simulink model "ROS_Control_for_ModularBus_cs"  (R2023a)
settings: Solver=ode5  StartTime=0.0  StopTime=inf  FixedStep=1/1000  RelTol=1e-3
PreLoadFcn:
  | mbxruntime.callbacks.PreLoadFcn(bdroot);
PostLoadFcn:
  | mbxruntime.callbacks.PostLoadFcn(bdroot);
InitFcn:
  | mbxruntime.callbacks.InitFcn(bdroot);
StartFcn:
  | mbxruntime.callbacks.StartFcn(bdroot);
StopFcn:
  | mbxruntime.callbacks.StopFcn(bdroot);
model workspace: external: MAT-File .\ROS_Control_for_ModularBus_cs_hws.mat (data not in the file)
values from neighbouring files (symbols this model uses):
  c_factor = 43.75    [emplanner_init.m]
  cf = -64276.3    [emplanner_init.m]
  cr = -64276.3    [emplanner_init.m]
  host_x_init = 0    [emplanner_init.m]
  host_y_init = 0    [emplanner_init.m]
  KD_PID_distance = 0.05    [emplanner_init.m]
  KD_PID_speed = 0.01    [emplanner_init.m]
  KI_PID_distance = 0.01    [emplanner_init.m]
  KI_PID_speed = 0.02    [emplanner_init.m]
  KP_PID_distance = 0.1    [emplanner_init.m]
  KP_PID_speed = 0.2    [emplanner_init.m]
  la = 0.5989    [emplanner_init.m]
  lb = 1.1979-0.5989    (= 0.599)    [emplanner_init.m]
  LQR_K1 = k(:,1)'    [emplanner_init.m]
  LQR_K2 = k(:,2)'    [emplanner_init.m]
  LQR_K3 = k(:,3)'    [emplanner_init.m]
  LQR_K4 = k(:,4)'    [emplanner_init.m]
  m = 375.8    [emplanner_init.m]
  vx_break_point = zeros(1,5000)    [emplanner_init.m]
undefined symbols (not defined in the file or in its folder): aubr, DiscIntNeverNeededParam, mbxruntime, rack_displacement, right_wheel_ground, ROS_Control_for_ModularBus_cs_018403cc6703814a, ROS_Control_for_ModularBus_cs_040a1db8f50ecaa9, ROS_Control_for_ModularBus_cs_059bdebef014cf08, ROS_Control_for_ModularBus_cs_0c250e3b2f70afe8, ROS_Control_for_ModularBus_cs_1665011a38ab79d0, ROS_Control_for_ModularBus_cs_17829354c8add7a7, ROS_Control_for_ModularBus_cs_19e468234ea448bc, ROS_Control_for_ModularBus_cs_27ae15b290bbaf4d, ROS_Control_for_ModularBus_cs_27eba31aa8e5b642, ROS_Control_for_ModularBus_cs_297ea4fdef143881, ROS_Control_for_ModularBus_cs_2b4063ae14d997a3, ROS_Control_for_ModularBus_cs_2c04773b04fadd8f, ROS_Control_for_ModularBus_cs_346eb3b7c82070b1, ROS_Control_for_ModularBus_cs_3f31df18790d0857, ROS_Control_for_ModularBus_cs_6035221df40a0068, ROS_Control_for_ModularBus_cs_605cc8a35cf1fbee, ROS_Control_for_ModularBus_cs_60f7501961f824af, ROS_Control_for_ModularBus_cs_6afca23e567ce192, ROS_Control_for_ModularBus_cs_722492775f672945, ROS_Control_for_ModularBus_cs_722a0847cfabd36b, ROS_Control_for_ModularBus_cs_739dd6601d79d035, ROS_Control_for_ModularBus_cs_7b4de5d0566f485f, ROS_Control_for_ModularBus_cs_7b8949829b72752d, ROS_Control_for_ModularBus_cs_82c4092e07cd044c, ROS_Control_for_ModularBus_cs_89fd7107669e07b9, ROS_Control_for_ModularBus_cs_8a6008cabae637b7, ROS_Control_for_ModularBus_cs_96f82902791ad622, ROS_Control_for_ModularBus_cs_9811c31d07ac9f2b, ROS_Control_for_ModularBus_cs_9ce2872cbf4b1b23, ROS_Control_for_ModularBus_cs_9d5a7f5c2803ee13, ROS_Control_for_ModularBus_cs_a623587393f1eaea, ROS_Control_for_ModularBus_cs_a7debeb2acd4f548, ROS_Control_for_ModularBus_cs_aa8fbbb7fdfec12a, ROS_Control_for_ModularBus_cs_ac425023a351a898, ROS_Control_for_ModularBus_cs_b3d4de7570946bb3, ROS_Control_for_ModularBus_cs_b771f0870c594399, ROS_Control_for_ModularBus_cs_bac30ea3d3bfebea, ROS_Control_for_ModularBus_cs_bd760ea296acac74, ROS_Control_for_ModularBus_cs_be4fa55e319672a9, ROS_Control_for_ModularBus_cs_c84eac9215852fa9, ROS_Control_for_ModularBus_cs_c9fa3144fa1cc4e3, ROS_Control_for_ModularBus_cs_caf32c655ee9484b, ROS_Control_for_ModularBus_cs_d133acedd44eb8df, ROS_Control_for_ModularBus_cs_d4613310abe0108f, ROS_Control_for_ModularBus_cs_dac9c98002987d8c, ROS_Control_for_ModularBus_cs_db335108f6550d72, ROS_Control_for_ModularBus_cs_dc60765170b71665, ROS_Control_for_ModularBus_cs_e0417f4e6fa341f5, ROS_Control_for_ModularBus_cs_e34124fd4d75bbae, ROS_Control_for_ModularBus_cs_e3fac3581a45c347, ROS_Control_for_ModularBus_cs_e5e08783dc4f74d5, ROS_Control_for_ModularBus_cs_ea1cf1e0b24b8a39, ROS_Control_for_ModularBus_cs_fa2a9ba8914f8ed6, ROS_Control_for_ModularBus_cs_faa52b96bad252bf, tablebr ... (+1)
libraries: PreScanSimulinkLibrary x18, robotlib x2, Solver_SF x1
(part 5 of 5)

== system ROS_Control_for_ModularBus_cs/Box_4/SELF_Demux/compas converter/cart2compas ==
  Angle [deg] : Inport
  Constant : Constant  Value=90
  Constant1 : Constant  Value=360
  Gain : Gain  Gain=1/360
  Gain1 : Gain  Gain=360
  Gain2 : Gain  Gain=-1
  Rounding Function : Rounding
  Sum : Sum  Inputs=|-+
  Sum1 : Sum  Inputs=-+|
  Sum2 : Sum  Inputs=++|
  heading [deg] : Outport
  wires:
  Gain/1 -> Rounding Function/1
  Rounding Function/1 -> Gain1/1
  Gain1/1 -> Sum/1
  Angle [deg]/1 -> Sum1/2
  Sum/1 -> Gain2/1
  Sum1/1 -> Gain/1, Sum/2
  Constant/1 -> Sum1/1
  Gain2/1 -> Sum2/2
  Constant1/1 -> Sum2/1
  Sum2/1 -> heading [deg]/1

== system ROS_Control_for_ModularBus_cs/Box_5/SELF_Demux/compas converter/cart2compas ==
  Angle [deg] : Inport
  Constant : Constant  Value=90
  Constant1 : Constant  Value=360
  Gain : Gain  Gain=1/360
  Gain1 : Gain  Gain=360
  Gain2 : Gain  Gain=-1
  Rounding Function : Rounding
  Sum : Sum  Inputs=|-+
  Sum1 : Sum  Inputs=-+|
  Sum2 : Sum  Inputs=++|
  heading [deg] : Outport
  wires:
  Gain/1 -> Rounding Function/1
  Rounding Function/1 -> Gain1/1
  Gain1/1 -> Sum/1
  Angle [deg]/1 -> Sum1/2
  Sum/1 -> Gain2/1
  Sum1/1 -> Gain/1, Sum/2
  Constant/1 -> Sum1/1
  Gain2/1 -> Sum2/2
  Constant1/1 -> Sum2/1
  Sum2/1 -> heading [deg]/1

== system ROS_Control_for_ModularBus_cs/Box_6/SELF_Demux/compas converter/cart2compas ==
  Angle [deg] : Inport
  Constant : Constant  Value=90
  Constant1 : Constant  Value=360
  Gain : Gain  Gain=1/360
  Gain1 : Gain  Gain=360
  Gain2 : Gain  Gain=-1
  Rounding Function : Rounding
  Sum : Sum  Inputs=|-+
  Sum1 : Sum  Inputs=-+|
  Sum2 : Sum  Inputs=++|
  heading [deg] : Outport
  wires:
  Gain/1 -> Rounding Function/1
  Rounding Function/1 -> Gain1/1
  Gain1/1 -> Sum/1
  Angle [deg]/1 -> Sum1/2
  Sum/1 -> Gain2/1
  Sum1/1 -> Gain/1, Sum/2
  Constant/1 -> Sum1/1
  Gain2/1 -> Sum2/2
  Constant1/1 -> Sum2/1
  Sum2/1 -> heading [deg]/1

== system ROS_Control_for_ModularBus_cs/Box_7/SELF_Demux/compas converter/cart2compas ==
  Angle [deg] : Inport
  Constant : Constant  Value=90
  Constant1 : Constant  Value=360
  Gain : Gain  Gain=1/360
  Gain1 : Gain  Gain=360
  Gain2 : Gain  Gain=-1
  Rounding Function : Rounding
  Sum : Sum  Inputs=|-+
  Sum1 : Sum  Inputs=-+|
  Sum2 : Sum  Inputs=++|
  heading [deg] : Outport
  wires:
  Gain/1 -> Rounding Function/1
  Rounding Function/1 -> Gain1/1
  Gain1/1 -> Sum/1
  Angle [deg]/1 -> Sum1/2
  Sum/1 -> Gain2/1
  Sum1/1 -> Gain/1, Sum/2
  Constant/1 -> Sum1/1
  Gain2/1 -> Sum2/2
  Constant1/1 -> Sum2/1
  Sum2/1 -> heading [deg]/1

== system ROS_Control_for_ModularBus_cs/Box_8/SELF_Demux/compas converter/cart2compas ==
  Angle [deg] : Inport
  Constant : Constant  Value=90
  Constant1 : Constant  Value=360
  Gain : Gain  Gain=1/360
  Gain1 : Gain  Gain=360
  Gain2 : Gain  Gain=-1
  Rounding Function : Rounding
  Sum : Sum  Inputs=|-+
  Sum1 : Sum  Inputs=-+|
  Sum2 : Sum  Inputs=++|
  heading [deg] : Outport
  wires:
  Gain/1 -> Rounding Function/1
  Rounding Function/1 -> Gain1/1
  Gain1/1 -> Sum/1
  Angle [deg]/1 -> Sum1/2
  Sum/1 -> Gain2/1
  Sum1/1 -> Gain/1, Sum/2
  Constant/1 -> Sum1/1
  Gain2/1 -> Sum2/2
  Constant1/1 -> Sum2/1
  Sum2/1 -> heading [deg]/1

== system ROS_Control_for_ModularBus_cs/modular_bus_1/Dynamics_UserSpecified/CarSim2PreScanSTATE/Transformation_SprungMassCarSim2PreScan ==
  In1 : Inport
  Demux : Demux  Outputs=3
  Ini z-position VEHICLE wrt GLOBAL axis system [m] : Constant  Value=z0
  Mux : Mux  Inputs=3
  Sum1 : Sum  Inputs=+-
  Out1 : Outport  VectorParamsAs1DForOutWhenUnconnected=off
  wires:
  Mux/1 -> Out1/1
  Ini z-position VEHICLE wrt GLOBAL axis system [m]/1 -> Sum1/2
  Demux/1 -> Mux/1
  Sum1/1 -> Mux/3
  Demux/3 -> Sum1/1
  Demux/2 -> Mux/2
  In1/1 -> Demux/1

== system ROS_Control_for_ModularBus_cs/modular_bus_1/SELF_Demux/compas converter/cart2compas ==
  Angle [deg] : Inport
  Constant : Constant  Value=90
  Constant1 : Constant  Value=360
  Gain : Gain  Gain=1/360
  Gain1 : Gain  Gain=360
  Gain2 : Gain  Gain=-1
  Rounding Function : Rounding
  Sum : Sum  Inputs=|-+
  Sum1 : Sum  Inputs=-+|
  Sum2 : Sum  Inputs=++|
  heading [deg] : Outport
  wires:
  Gain/1 -> Rounding Function/1
  Rounding Function/1 -> Gain1/1
  Gain1/1 -> Sum/1
  Angle [deg]/1 -> Sum1/2
  Sum/1 -> Gain2/1
  Sum1/1 -> Gain/1, Sum/2
  Constant/1 -> Sum1/1
  Gain2/1 -> Sum2/2
  Constant1/1 -> Sum2/1
  Sum2/1 -> heading [deg]/1

== system ROS_Control_for_ModularBus_cs/modular_bus_1/control module/control main/chassic steering system ==
  LQR_final_angle : Inport
  Constant : Constant  Value=la
  Constant1 : Constant  Value=lb
  Constant17 : Constant  Value=c_factor
  Divide : Product  Inputs=*/
  Gain3 : Gain  Gain=180/pi
  Gain4 : Gain  Gain=360
  MATLAB Function : MATLAB Function  TreatAsAtomicUnit=on
  Saturation : Saturate  UpperLimit=70  LowerLimit=-70
  Saturation1 : Saturate  UpperLimit=1.2217  LowerLimit=-1.2217
  transfer right wheel angle to rack displancement : Lookup_n-D  NumberOfTableDimensions=1  BreakpointsForDimension1=right_wheel_ground  Table=rack_displacement  InternalRulePriority=Speed  RndMeth=Simplest
  lat_steer_sw[deg] : Outport
  wires:
  transfer right wheel angle to rack displancement/1 -> Divide/1
  Constant17/1 -> Divide/2
  Gain4/1 -> lat_steer_sw[deg]/1
  Divide/1 -> Gain4/1
  Saturation/1 -> transfer right wheel angle to rack displancement/1
  Constant/1 -> MATLAB Function/2(la)
  Gain3/1 -> Saturation/1
  Constant1/1 -> MATLAB Function/3(lb)
  LQR_final_angle/1 -> Saturation1/1
  Saturation1/1 -> MATLAB Function/1(u)
  MATLAB Function/1(right_steer) -> Gain3/1

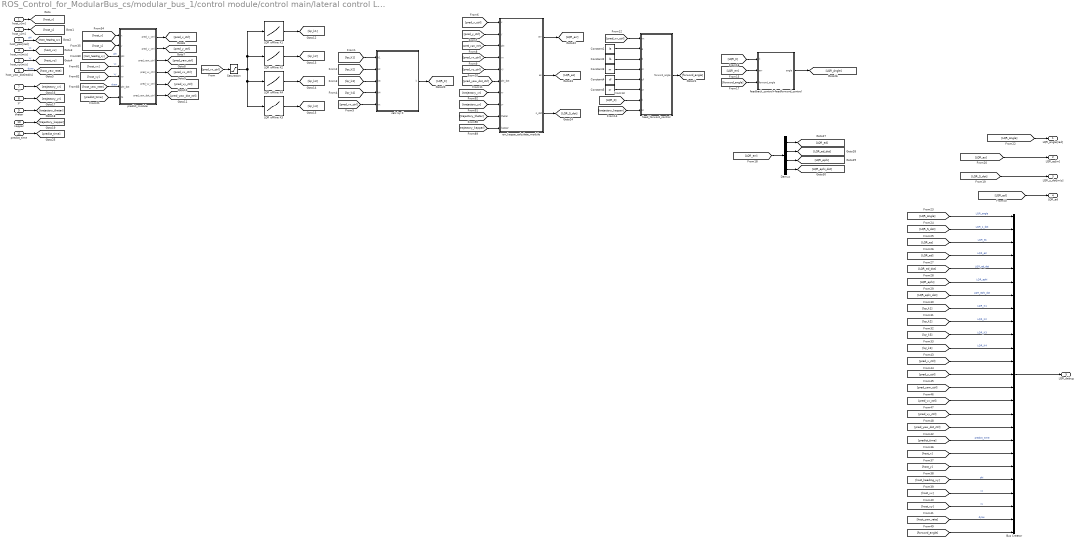
== system ROS_Control_for_ModularBus_cs/modular_bus_1/control module/control main/lateral control LQR ==
  host_x[m] : Inport
  host_y[m] : Inport  Port=2
  host_yaw[rad] : Inport  Port=3
  host_vx[m/s] : Inport  Port=4
  host_vy[m/s] : Inport  Port=5
  host_yaw_dot[rad/s] : Inport  Port=6
  xr : Inport  Port=7
  yr : Inport  Port=8
  thetar : Inport  Port=9
  kappar : Inport  Port=10
  predict_time : Inport  Port=11
  Bus Creator : BusCreator  Inputs=25
  Constant1 : Constant  Value=la
  Constant2 : Constant  Value=lb
  Constant3 : Constant  Value=m
  Constant4 : Constant  Value=cf
  Constant5 : Constant  Value=cr
  Demux : Demux
  LQR offline K1 : Lookup_n-D  NumberOfTableDimensions=1  BreakpointsForDimension1=vx_break_point  Table=LQR_K1  InternalRulePriority=Speed  RndMeth=Simplest
  LQR offline K2 : Lookup_n-D  NumberOfTableDimensions=1  BreakpointsForDimension1=vx_break_point  Table=LQR_K2  InternalRulePriority=Speed  RndMeth=Simplest
  LQR offline K3 : Lookup_n-D  NumberOfTableDimensions=1  BreakpointsForDimension1=vx_break_point  Table=LQR_K3  InternalRulePriority=Speed  RndMeth=Simplest
  LQR offline K4 : Lookup_n-D  NumberOfTableDimensions=1  BreakpointsForDimension1=vx_break_point  Table=LQR_K4  InternalRulePriority=Speed  RndMeth=Simplest
  Saturation : Saturate  UpperLimit=50  LowerLimit=0
  calc lqr K : MATLAB Function  TreatAsAtomicUnit=on
  err_kappa_calculate_module : MATLAB Function  TreatAsAtomicUnit=on
  feed_forword_control : MATLAB Function  TreatAsAtomicUnit=on
  feedback_control+feedforword_control : MATLAB Function  TreatAsAtomicUnit=on
  predict_module : MATLAB Function  TreatAsAtomicUnit=on
  LQR_angle[rad] : Outport  VectorParamsAs1DForOutWhenUnconnected=off
  LQR_es[m] : Outport  Port=2  VectorParamsAs1DForOutWhenUnconnected=off
  LQR_s_dot[m/s] : Outport  Port=3  VectorParamsAs1DForOutWhenUnconnected=off
  LQR_ed : Outport  Port=4  VectorParamsAs1DForOutWhenUnconnected=off
  LQR_debug : Outport  Port=5  VectorParamsAs1DForOutWhenUnconnected=off
  wires:
  [host_vy] -> predict_module/5(vy)  "vy"
  [host_x] -> predict_module/1(x)
  [host_yaw_rate] -> predict_module/6(phi_dot)  "dyaw"
  [host_vx] -> predict_module/4(vx)  "vx"
  [host_y] -> predict_module/2(y)
  [host_heading_xy] -> predict_module/3(phi)  "phi"
  [predict_time] -> predict_module/7(ts)
  host_x[m]/1 -> [host_x]
  host_y[m]/1 -> [host_y]
  host_yaw[rad]/1 -> [host_heading_xy]  "phi"
  host_vx[m/s]/1 -> [host_vx]  "vx"
  host_vy[m/s]/1 -> [host_vy]  "vy"
  host_yaw_dot[rad/s]/1 -> [host_yaw_rate]  "dyaw"
  predict_module/1(pred_x_ctrl) -> [pred_x_ctrl]
  predict_module/2(pred_y_ctrl) -> [pred_y_ctrl]
  predict_module/3(pred_yaw_ctrl) -> [pred_yaw_ctrl]
  predict_module/4(pred_vx_ctrl) -> [pred_vx_ctrl]
  predict_module/5(pred_vy_ctrl) -> [pred_vy_ctrl]
  predict_module/6(pred_yaw_dot_ctrl) -> [pred_yaw_dot_ctrl]
  [pred_vx_ctrl] -> Saturation/1
  LQR offline K1/1 -> [lqr_k1]
  LQR offline K2/1 -> [lqr_k2]
  LQR offline K4/1 -> [lqr_k3]
  LQR offline K3/1 -> [lqr_k4]
  [pred_vx_ctrl] -> calc lqr K/5(vx)
  [lqr_k4] -> calc lqr K/4(k4)
  [lqr_k3] -> calc lqr K/3(k3)
  [lqr_k2] -> calc lqr K/2(k2)
  [lqr_k1] -> calc lqr K/1(k1)
  [pred_x_ctrl] -> err_kappa_calculate_module/1(x)
  [pred_y_ctrl] -> err_kappa_calculate_module/2(y)
  [pred_yaw_ctrl] -> err_kappa_calculate_module/3(phi)
  [pred_vx_ctrl] -> err_kappa_calculate_module/4(vx)
  [pred_vy_ctrl] -> err_kappa_calculate_module/5(vy)
  [pred_yaw_dot_ctrl] -> err_kappa_calculate_module/6(phi_dot)
  xr/1 -> [trajectory_xr]
  yr/1 -> [trajectory_yr]
  thetar/1 -> [trajectory_thetar]
  kappar/1 -> [trajectory_kappar]
  [trajectory_xr] -> err_kappa_calculate_module/7(xr)
  [trajectory_yr] -> err_kappa_calculate_module/8(yr)
  [trajectory_kappar] -> err_kappa_calculate_module/10(kappar)
  [trajectory_thetar] -> err_kappa_calculate_module/9(thetar)
  [pred_vx_ctrl] -> feed_forword_control/1(vx)
  Constant1/1 -> feed_forword_control/2(a)
  Constant2/1 -> feed_forword_control/3(b)
  Constant3/1 -> feed_forword_control/4(m)
  Constant4/1 -> feed_forword_control/5(cf)
  Constant5/1 -> feed_forword_control/6(cr)
  calc lqr K/1(k) -> [LQR_K]
  [LQR_K] -> feed_forword_control/7(k)
  [trajectory_kappar] -> feed_forword_control/8(kr)
  feed_forword_control/1(forword_angle) -> [forword_angle]
  err_kappa_calculate_module/1(err) -> [LQR_err]
  [LQR_err] -> feedback_control+feedforword_control/2(err)
  [LQR_K] -> feedback_control+feedforword_control/1(k)
  [forword_angle] -> feedback_control+feedforword_control/3(forword_angle)
  [LQR_err] -> Demux/1
  err_kappa_calculate_module/2(es) -> [LQR_es]
  err_kappa_calculate_module/3(s_dot) -> [LQR_S_dot]
  [LQR_S_dot] -> LQR_s_dot[m/s]/1
  [LQR_es] -> LQR_es[m]/1
  Saturation/1 -> LQR offline K3/1, LQR offline K4/1, LQR offline K2/1, LQR offline K1/1
  predict_time/1 -> [predict_time]
  Bus Creator/1 -> LQR_debug/1
  feedback_control+feedforword_control/1(angle) -> [LQR_Angle]
  [LQR_Angle] -> LQR_angle[rad]/1
  [LQR_Angle] -> Bus Creator/1  "LQR_angle"
  [LQR_S_dot] -> Bus Creator/2  "LQR_s_dot"
  [LQR_es] -> Bus Creator/3  "LQR_es"
  Demux/1 -> [LQR_ed]
  Demux/2 -> [LQR_ed_dot]
  Demux/3 -> [LQR_ephi]
  Demux/4 -> [LQR_ephi_dot]
  [LQR_ed] -> Bus Creator/4  "LQR_ed"
  [LQR_ed_dot] -> Bus Creator/5  "LQR_ed_dot"
  [LQR_ephi] -> Bus Creator/6  "LQR_ephi"
  [LQR_ephi_dot] -> Bus Creator/7  "LQR_ephi_dot"
  [lqr_k1] -> Bus Creator/8  "LQR_K1"
  [lqr_k2] -> Bus Creator/9  "LQR_K2"
  [lqr_k3] -> Bus Creator/10  "LQR_K3"
  [lqr_k4] -> Bus Creator/11  "LQR_K4"
  [pred_x_ctrl] -> Bus Creator/12
  [pred_y_ctrl] -> Bus Creator/13
  [pred_yaw_ctrl] -> Bus Creator/14
  [pred_vx_ctrl] -> Bus Creator/15
  [pred_vy_ctrl] -> Bus Creator/16
  [pred_yaw_dot_ctrl] -> Bus Creator/17
  [predict_time] -> Bus Creator/18  "predict_time"
  [host_x] -> Bus Creator/19
  [host_y] -> Bus Creator/20
  [host_heading_xy] -> Bus Creator/21  "phi"
  [host_vx] -> Bus Creator/22  "vx"
  [host_vy] -> Bus Creator/23  "vy"
  [host_yaw_rate] -> Bus Creator/24  "dyaw"
  [forword_angle] -> Bus Creator/25
  [LQR_ed] -> LQR_ed/1

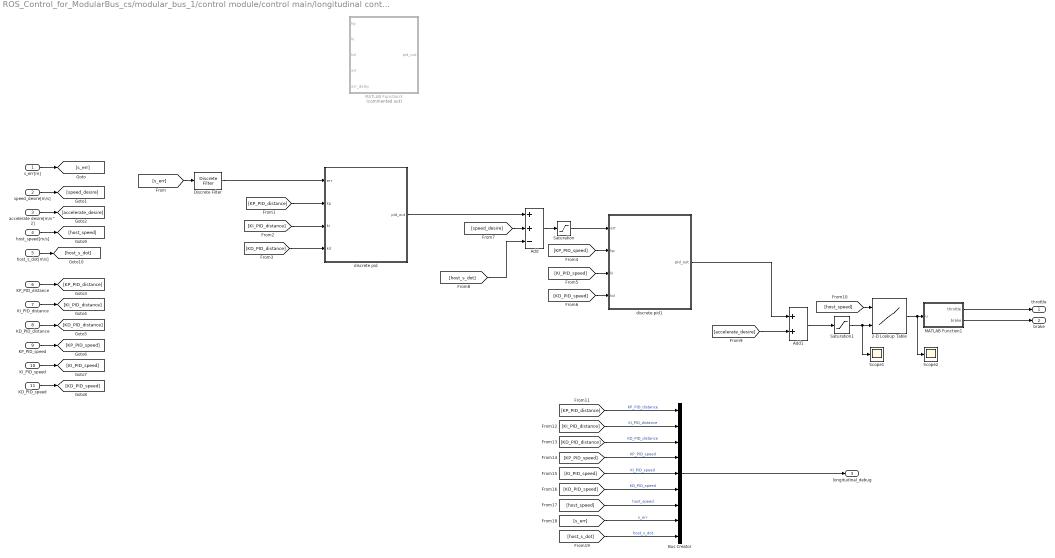
== system ROS_Control_for_ModularBus_cs/modular_bus_1/control module/control main/longitudinal control double PID ==
  s_err[m] : Inport
  speed_desire[m/s] : Inport  Port=2
  accelerate desire[m/s^2] : Inport  Port=3
  host_speed[m/s] : Inport  Port=4
  host_s_dot[m/s] : Inport  Port=5
  KP_PID_distance : Inport  Port=6
  KI_PID_distance : Inport  Port=7
  KD_PID_distance : Inport  Port=8
  KP_PID_speed : Inport  Port=9
  KI_PID_speed : Inport  Port=10
  KD_PID_speed : Inport  Port=11
  2-D Lookup Table : Lookup_n-D  BreakpointsForDimension1=vubr  BreakpointsForDimension2=aubr  Table=tablebr  InternalRulePriority=Speed  RndMeth=Simplest
      settings: InputPortMap=u0,u1
  Add : Sum  Inputs=++-
  Add1 : Sum
  Bus Creator : BusCreator  Inputs=9
  Discrete Filter : DiscreteFilter
  MATLAB Function1 : MATLAB Function  TreatAsAtomicUnit=on
  MATLAB Function3 : MATLAB Function  Commented=on  TreatAsAtomicUnit=on
  Saturation : Saturate  UpperLimit=45  LowerLimit=-45
  Saturation1 : Saturate  UpperLimit=5  LowerLimit=-8
  Scope1 : Scope
  Scope2 : Scope
  discrete pid : Subsystem
  discrete pid1 : Subsystem
  throttle : Outport
  brake : Outport  Port=2
  longitudinal_debug : Outport  Port=3
  wires:
  2-D Lookup Table/1 -> Scope2/1, MATLAB Function1/1(u)
  s_err[m]/1 -> [s_err]
  speed_desire[m/s]/1 -> [speed_desire]
  accelerate desire[m/s^2]/1 -> [accelerate_desire]
  KP_PID_distance/1 -> [KP_PID_distance]
  KI_PID_distance/1 -> [KI_PID_distance]
  KD_PID_distance/1 -> [KD_PID_distance]
  KP_PID_speed/1 -> [KP_PID_speed]
  KI_PID_speed/1 -> [KI_PID_speed]
  KD_PID_speed/1 -> [KD_PID_speed]
  [s_err] -> Discrete Filter/1
  host_speed[m/s]/1 -> [host_speed]
  [speed_desire] -> Add/2
  Add/1 -> Saturation/1
  Saturation/1 -> discrete pid1/1(err)
  discrete pid1/1(pid_out) -> Add1/1
  [accelerate_desire] -> Add1/2
  Add1/1 -> Saturation1/1
  Saturation1/1 -> Scope1/1, 2-D Lookup Table/2
  host_s_dot[m/s]/1 -> [host_s_dot]
  [host_s_dot] -> Add/3
  [host_speed] -> 2-D Lookup Table/1
  MATLAB Function1/1(throttle) -> throttle/1
  MATLAB Function1/2(brake) -> brake/1
  [KP_PID_distance] -> Bus Creator/1  "KP_PID_distance"
  [KI_PID_distance] -> Bus Creator/2  "KI_PID_distance"
  [KD_PID_distance] -> Bus Creator/3  "KD_PID_distance"
  [KP_PID_speed] -> Bus Creator/4  "KP_PID_speed"
  [KI_PID_speed] -> Bus Creator/5  "KI_PID_speed"
  [KD_PID_speed] -> Bus Creator/6  "KD_PID_speed"
  [host_speed] -> Bus Creator/7  "host_speed"
  [s_err] -> Bus Creator/8  "s_err"
  [host_s_dot] -> Bus Creator/9  "host_s_dot"
  Bus Creator/1 -> longitudinal_debug/1
  discrete pid/1(pid_out) -> Add/1
  Discrete Filter/1 -> discrete pid/1(err)
  [KP_PID_distance] -> discrete pid/2(kp)
  [KI_PID_distance] -> discrete pid/3(ki)
  [KD_PID_distance] -> discrete pid/4(kd)
  [KP_PID_speed] -> discrete pid1/2(kp)
  [KI_PID_speed] -> discrete pid1/3(ki)
  [KD_PID_speed] -> discrete pid1/4(kd)

== system ROS_Control_for_ModularBus_cs/modular_bus_1/control module/control main/understeer compensate ==
  LQR_angle : Inport
  lateral err : Inport  Port=2
  Add : Sum  Inputs=+-
  Gain : Gain  Gain=0.01
  Manual Switch : ManualSwitch
  LQR_final_angle : Outport
  wires:
  lateral err/1 -> Gain/1
  Add/1 -> Manual Switch/2
  Manual Switch/1 -> LQR_final_angle/1
  LQR_angle/1 -> Add/1, Manual Switch/1
  Gain/1 -> Add/2

== system ROS_Control_for_ModularBus_cs/modular_bus_1/control module/control main/longitudinal control double PID/discrete pid ==
  err : Inport
  kp : Inport  Port=2
  ki : Inport  Port=3
  kd : Inport  Port=4
  Add2 : Sum  Inputs=+++
  Add3 : Sum
  Add4 : Sum  Inputs=+-
  Delay3 : Delay  DelayLength=1
  Delay4 : Delay  DelayLength=1
  Divide : Product  Inputs=**
  Divide1 : Product  Inputs=**
  Divide2 : Product  Inputs=**
  Gain : Gain  Gain=0.01
  pid_out : Outport
  wires:
  [KD_PID_distance] -> Divide2/2
  err/1 -> Delay4/1, Divide/2, Add3/1, Add4/1
  Divide/1 -> Add2/1
  Divide2/1 -> Add2/3
  Add3/1 -> Gain/1, Divide1/1
  Delay4/1 -> Add4/2
  [KP_PID_distance] -> Divide/1
  Divide1/1 -> Add2/2
  Delay3/1 -> Add3/2
  [KI_PID_distance] -> Divide1/2
  Add4/1 -> Divide2/1
  Add2/1 -> pid_out/1
  kp/1 -> [KP_PID_distance]
  ki/1 -> [KI_PID_distance]
  kd/1 -> [KD_PID_distance]
  Gain/1 -> Delay3/1

== system ROS_Control_for_ModularBus_cs/modular_bus_1/control module/control main/longitudinal control double PID/discrete pid1 ==
  err : Inport
  kp : Inport  Port=2
  ki : Inport  Port=3
  kd : Inport  Port=4
  Add2 : Sum  Inputs=+++
  Add3 : Sum
  Add4 : Sum  Inputs=+-
  Delay3 : Delay  DelayLength=1
  Delay4 : Delay  DelayLength=1
  Divide : Product  Inputs=**
  Divide1 : Product  Inputs=**
  Divide2 : Product  Inputs=**
  Gain : Gain  Gain=0.01
  pid_out : Outport
  wires:
  Gain/1 -> Delay3/1
  kd/1 -> [KD_PID_distance]
  ki/1 -> [KI_PID_distance]
  kp/1 -> [KP_PID_distance]
  Add2/1 -> pid_out/1
  Add4/1 -> Divide2/1
  [KI_PID_distance] -> Divide1/2
  Delay3/1 -> Add3/2
  Divide1/1 -> Add2/2
  [KP_PID_distance] -> Divide/1
  Delay4/1 -> Add4/2
  Add3/1 -> Divide1/1, Gain/1
  Divide2/1 -> Add2/3
  Divide/1 -> Add2/1
  err/1 -> Add4/1, Add3/1, Divide/2, Delay4/1
  [KD_PID_distance] -> Divide2/2

== matlab function ROS_Control_for_ModularBus_cs/modular_bus_1/control module/control main/lateral control LQR/feed_forword_control ==
  data: vx input; a input; forword_angle output; b input; m input; cf input; cr input; k input; kr input
function forword_angle = fcn(vx,a,b,m,cf,cr,k,kr)
    forword_angle=kr*(a+b-b*k(3)-(m*vx*vx/(a+b))*((b/cf)+(a/cr)*k(3)-(a/cr)));
end

== matlab function ROS_Control_for_ModularBus_cs/modular_bus_1/control module/control main/lateral control LQR/feedback_control+feedforword_control ==
  data: k input; angle output; err input; forword_angle input
function angle = fcn(k,err,forword_angle)

    angle=-k*err+forword_angle;
end

== matlab function ROS_Control_for_ModularBus_cs/modular_bus_1/control module/control main/lateral control LQR/calc lqr K ==
  data: k1 input; k output; k2 input; k3 input; k4 input; vx input
function k  = fcn(k1,k2,k3,k4,vx)
    if abs(vx)<0.1
        k=[0,0,0,0];
    else
       
        k=[k1,k2,k3,k4];
    end
end

== matlab function ROS_Control_for_ModularBus_cs/modular_bus_1/control module/control main/lateral control LQR/predict_module ==
  data: x input; pred_x_ctrl output; y input; phi input; vx input; vy input; phi_dot input; ts input; pred_y_ctrl output; pred_yaw_ctrl output; pred_vx_ctrl output; pred_vy_ctrl output; pred_yaw_dot_ctrl output
function [pred_x_ctrl,pred_y_ctrl,pred_yaw_ctrl,pred_vx_ctrl,pred_vy_ctrl,pred_yaw_dot_ctrl] = fcn(x,y,phi,vx,vy,phi_dot,ts)
    pred_x_ctrl=x+vx*ts*cos(phi)-vy*ts*sin(phi);
    pred_y_ctrl=y+vy*ts*cos(phi)+vx*ts*sin(phi);
    pred_yaw_ctrl=phi;
    pred_vx_ctrl=vx;
    pred_vy_ctrl=vy;
    pred_yaw_dot_ctrl=phi_dot;
end

== matlab function ROS_Control_for_ModularBus_cs/modular_bus_1/control module/control main/chassic steering system/MATLAB Function ==
  data: u input; right_steer output; la input; lb input
function right_steer = fcn(u,la,lb)
if abs(u)<1e-2
   right_steer = u;
else
   R =  (la+lb)/tan(u);
   right_steer = atan((la+lb)/(R+1.624/2));
end

== stateflow chart ROS_Control_for_ModularBus_cs/modular_bus_1/Schedule OS ==
  (default) -> (junction 5)
  (junction 5) -> (junction 9) [order 1] : [i>100]
  (junction 5) -> (junction 10) [order 2] : {i = i+1;}
  (junction 9) -> (junction 12) : {
      | do_planning;
      | i = 0;
      | }
  (junction 12) -> (junction 10)
  (junction 10) -> (junction 15)
  (junction 15) -> (junction 17) [order 1] : [j>10]
  (junction 15) -> (junction 21) [order 2] : {j = j+1}
  (junction 17) -> (junction 19) : {
      | do_control;
      | j = 0;
      | }
  (junction 19) -> (junction 21)
  (junction 21) -> (junction 24)
  data: i local =1; j local =1
  events: do_planning output FUNCTION_CALL_EVENT; do_control output FUNCTION_CALL_EVENT

== matlab function ROS_Control_for_ModularBus_cs/modular_bus_1/planning module/test planning ==
  data: xr output; yr output; thetar output; kr output; t input; vp output; ap output; x_init input; y_init input
function [xr,yr,thetar,kr,vp,ap] = fcn(t,x_init,y_init)
    dx=100;
    dy=10;
    T=30;
    xstart=[x_init,0,0];
    xend=[dx+x_init,0,0];
    ystart=[y_init,0,0];
    yend=[dy+y_init,0,0];
    a=zeros(1,6);
    b=zeros(1,6);
    
    a(1)=xstart(1);
    a(2)=xstart(2);
    a(3)=xstart(3)/2;
    A1=[T^3,T^4,T^5;
        3*T^2,4*T^3,5*T^4;
        6*T,12*T^2,20*T^3];
    B1=[xend(1)-a(1)-a(2)*T-a(3)*T^2;
        xend(2)-a(2)-2*a(3)*T;
        xend(3)-2*a(3)];
    xs=inv(A1)*B1;
    a(4)=xs(1);
    a(5)=xs(2);
    a(6)=xs(3);
    b(1)=ystart(1);
    b(2)=ystart(2);
    b(3)=ystart(3)/2;
    A2=[dx^3,dx^4,dx^5;
        3*dx^2,4*dx^3,5*dx^4;
        6*dx,12*dx^2,20*dx^3];
    B2=[yend(1)-b(1)-b(2)*dx-b(3)*dx^2;
        yend(2)-b(2)-2*b(3)*dx;
        yend(3)-2*b(3)];
    ys=inv(A2)*B2;
    b(4)=ys(1);
    b(5)=ys(2);
    b(6)=ys(3);
    xr=a(1)+a(2)*t+a(3)*t^2+a(4)*t^3+a(5)*t^4+a(6)*t^5;
    yr=b(1)+b(2)*xr+b(3)*xr^2+b(4)*xr^3+b(5)*xr^4+b(6)*xr^5;
    xr_dot=a(2)+2*a(3)*t+3*a(4)*t^2+4*a(5)*t^3+5*a(6)*t^4;
    yr_dx=b(2)+2*b(3)*xr+3*b(4)*xr^2+4*b(5)*xr^3+5*b(6)*xr^4;
    yr_dot=yr_dx*xr_dot;
    thetar=atan(yr_dx);
    xr_dot2=2*a(3)+6*a(4)*t+12*a(5)*t^2+20*a(6)*t^3;
    yr_dx2=2*b(3)+6*b(4)*xr+12*b(5)*xr^2+20*b(6)*xr^3;
    yr_dot2=yr_dx2*xr_dot^2+yr_dx*xr_dot2;
    kr=yr_dx2/((1+yr_dx^2)^1.5);
    vp=sqrt(xr_dot^2+yr_dot^2);
    if xr_dot2>=0
        ap=sqrt(xr_dot2^2+yr_dot2^2);
    else
        ap=-sqrt(xr_dot2^2+yr_dot2^2);
    end

== matlab function ROS_Control_for_ModularBus_cs/modular_bus_1/control module/control main/longitudinal control double PID/MATLAB Function1 ==
  data: u input; throttle output; brake output
function [throttle,brake] = fcn(u)
    if u>=0
        throttle=u;
        brake=0;
    else
        throttle=0;
        brake=-u;
    end

== matlab function ROS_Control_for_ModularBus_cs/modular_bus_1/control module/control main/longitudinal control double PID/MATLAB Function3 ==
  data: kp input; pid_out output; ki input; kd input; err input; err_delay input
function pid_out = fcn(kp,ki,kd,err,err_delay)

persistent integral;
if isempty(integral)
    integral = err * ki *0.01;
    devia = kd*(err - err_delay)/0.01;
    pid_out = kp*err + integral + devia;
else
    integral = integral + err * ki *0.01;
    devia = kd*(err - err_delay)/0.01;
    pid_out = kp*err + integral + devia;
end

== matlab function ROS_Control_for_ModularBus_cs/modular_bus_1/control module/control main/lateral control LQR/err_kappa_calculate_module ==
  data: x input; y input; phi input; vx input; vy input; phi_dot input; xr input; yr input; thetar input; kappar input; err output; es output; s_dot output
function [err,es,s_dot] = fcn(x,y,phi,vx,vy,phi_dot,xr,yr,thetar,kappar)
    
    tor=[cos(thetar);sin(thetar)];
    nor=[-sin(thetar);cos(thetar)];
    d_err=[x-xr;y-yr];
    ed=nor'*d_err;
    es=tor'*d_err;
    %projection_point_thetar=thetar(dmin);%apollo
    projection_point_thetar=thetar+kappar*es;
    ed_dot=vy*cos(phi-projection_point_thetar)+vx*sin(phi-projection_point_thetar);
    %%%%%%%%%
    ephi=sin(phi-projection_point_thetar);
    %%%%%%%%%
    ss_dot=vx*cos(phi-projection_point_thetar)-vy*sin(phi-projection_point_thetar);
    s_dot=ss_dot/(1-kappar*ed);
    ephi_dot=phi_dot-kappar*s_dot;
    err=[ed;ed_dot;ephi;ephi_dot];
    
    
    
    
    
    
    
    
    
    
    
    


end
